simulink library "miniview_lib"  (Simulink 5.1)
undefined symbols (not defined in the file or in its folder): DN, miniview_string_xfer_page0, miniview_string_xfer_page1, miniview_string_xfer_page2, ptr, UP
libraries: simulink x33, MotoHawk_lib x17, miniview_lib x8
settings Model: LastModifiedBy=Chris_Doyle  ProdHWDeviceType=Microprocessor

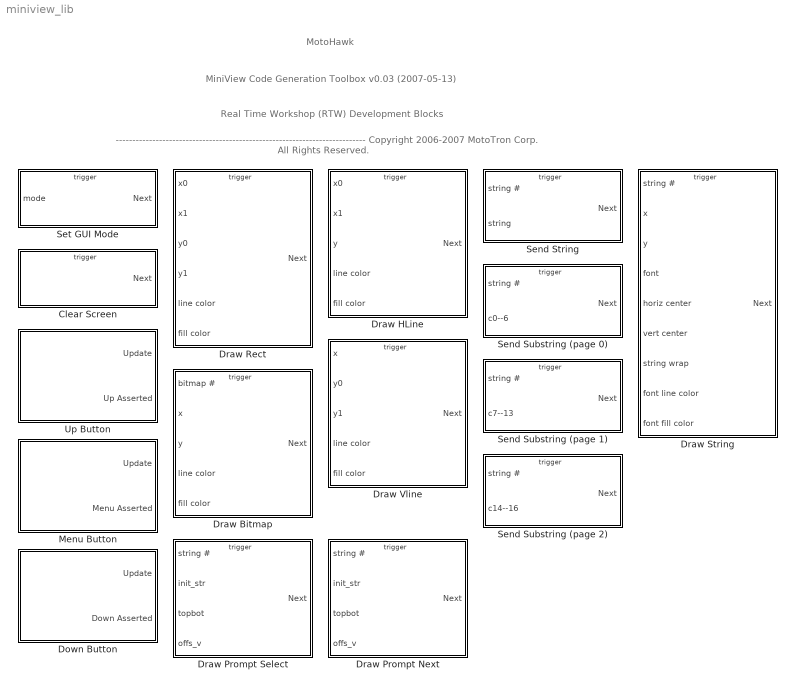
== system miniview_lib ==
  note: MotoHawk
  note: ---------------------------------------------------------------------------
      | Copyright 2006-2007 MotoTron Corp.  All Rights Reserved.
  note: Real Time Workshop (RTW)
      | Development Blocks
  note: MiniView Code Generation Toolbox v0.03 (2007-05-13)
  Clear Screen : Subsystem  mask(MotoHawk MiniView Clear Screen){miniview_CAN_channel=2}
      mask prompts: miniview_CAN_channel "Physical CAN Channel"
      mask help: MotoHawk MiniView Clear Screen
      mask Display: disp(['\nMiniView\nClear Screen\nChannel:  CAN_' num2str(miniview_CAN_channel)])
  Down Button : Subsystem  mask(MotoHawk MiniView Down Button){miniview_CAN_channel=2}
      mask prompts: miniview_CAN_channel "Physical CAN Channel"
      mask help: MotoHawk MiniView Down Button
      mask Display: disp(['MiniView "Down" Button\nChannel:  CAN_' num2str(miniview_CAN_channel)])
  Draw Bitmap : Subsystem  mask(MotoHawk MiniView Draw Bitmap){miniview_CAN_channel=2}
      mask prompts: miniview_CAN_channel "Physical CAN Channel"
      mask help:
      | MotoHawk MiniView Draw Bitmap
      | 0:  "Dialog"
      | 1:  small down-arrow
      | 2:  large down-arrow
      | 3:  selector down-arrow
      | 4:  selector up-arrow
      mask Display: disp(['MiniView\nDraw Bitmap\nChannel:  CAN_' num2str(miniview_CAN_channel) '\n\n\n\n'])
  Draw HLine : Subsystem  mask(MotoHawk MiniView Draw Horizontal Line){miniview_CAN_channel=2}
      mask prompts: miniview_CAN_channel "Physical CAN Channel"
      mask help: MotoHawk MiniView Draw Horizontal Line
      mask Display: disp(['MiniView\nDraw Horiz Line\nChannel:  CAN_' num2str(miniview_CAN_channel) '\n\n\n\n'])
  Draw Prompt Next : Subsystem  mask(MotoHawk MiniView Draw Prompt Next){miniview_CAN_channel=2}
      mask prompts: miniview_CAN_channel "Physical CAN Channel"
      mask help:
      | MotoHawk MiniView Draw Prompt Next
      |
      | string # (0 to 15):  which string buffer to use.
      |
      | init_str (F,T):  when TRUE, initialize string buffer in gauge (by sending CAN message).  must be done first time prompt is drawn, and whenever buffer has been changed.
      |
      | topbot (F,T):  when FALSE, prompt at "top" position; when TRUE, prompt at "bottom" position.
      |
      | offs_v (0 to 55 when topbot is FALSE, otherwise 0):  vertical offset (downwards) for prompt from "top" position.
      mask Display: disp(['\nDraw\nPrompt\n[up]NEXT[dn]\nChannel:  CAN_' num2str(miniview_CAN_channel)])
  Draw Prompt Select : Subsystem  mask(MotoHawk MiniView Draw Prompt Select){miniview_CAN_channel=2}
      mask prompts: miniview_CAN_channel "Physical CAN Channel"
      mask help:
      | MotoHawk MiniView Draw Prompt Select
      |
      | string # (0 to 15):  which string buffer to use.
      |
      | init_str (F,T):  when TRUE, initialize string buffer in gauge (by sending CAN message).  must be done first time prompt is drawn, and whenever buffer has been changed.
      |
      | topbot (F,T):  when FALSE, prompt at "top" position; when TRUE, prompt at "bottom" position.
      |
      | offs_v (0 to 55 when topbot is FALSE, otherwise 0):  vertical offset (downwards) for prompt from "top" position.
      mask Display: disp(['\nDraw\nPrompt\n[up]SEL[dn]\nChannel:  CAN_' num2str(miniview_CAN_channel)])
  Draw Rect : Subsystem  mask(MotoHawk MiniView Draw Rectangle){miniview_CAN_channel=2}
      mask prompts: miniview_CAN_channel "Physical CAN Channel"
      mask help: MotoHawk MiniView Draw Rectangle
      mask Display: disp(['MiniView\nDraw Rectangle\nChannel:  CAN_' num2str(miniview_CAN_channel) '\n\n\n\n'])
  Draw String : Subsystem  mask(MotoHawk MiniView Draw String){miniview_CAN_channel=2}
      mask prompts: miniview_CAN_channel "Physical CAN Channel"
      mask help:
      | MotoHawk MiniView Draw String
      |
      | Draw string (#0 to #15) previously sent to gauge using "Send String"
      | or "Send Substring (Page 0/1/2)" blocks.
      |
      | Comment:  "Font Fill Color" input is ignored.
      mask Display: disp(['MiniView\nDraw String\nChannel:  CAN_' num2str(miniview_CAN_channel) '\n\n\n\n'])
  Draw Vline : Subsystem  mask(MotoHawk MiniView Draw Vertical Line){miniview_CAN_channel=2}
      mask prompts: miniview_CAN_channel "Physical CAN Channel"
      mask help: MotoHawk MiniView Draw Vertical Line
      mask Display: disp(['MiniView\nDraw Vert Line\nChannel:  CAN_' num2str(miniview_CAN_channel) '\n\n\n\n'])
  Menu Button : Subsystem  mask(MotoHawk MiniView Menu Button){miniview_CAN_channel=2}
      mask prompts: miniview_CAN_channel "Physical CAN Channel"
      mask help: MotoHawk MiniView Menu Button
      mask Display: disp(['MiniView "Menu" Button\nChannel:  CAN_' num2str(miniview_CAN_channel)])
  Send String : Subsystem  mask(MotoHawk MiniView Send String){miniview_CAN_channel=2}
      mask prompts: miniview_CAN_channel "Physical CAN Channel"
      mask help:
      | MotoHawk MiniView Send String
      |
      | Send string (#0 to #15) to gauge.
      mask Display: disp(['MiniView\nSend String\nChannel:  CAN_' num2str(miniview_CAN_channel)])
  Send Substring (page 0) : Subsystem  mask(MotoHawk MiniView Send String (Page 0)){miniview_CAN_channel=2}
      mask prompts: miniview_CAN_channel "Physical CAN Channel"
      mask help:
      | MotoHawk MiniView Send String (Page 0)
      |
      | Send first seven characters (0 to 6) of string (#0 to #15) to gauge.
      |
      | Before using a string, all three pages (0/1/2) must be sent using either "Send String" block to send the entire string at once, or by sending each page using "Send Substring (Page 0/1/2)" blocks.
      |
      | The "Send Substring (Page 0/1/2)" blocks may also be used to modify a previously-sent string.
      mask Display: disp(['MiniView\nSend Substr Pg 0\nChannel:  CAN_' num2str(miniview_CAN_channel)])
  Send Substring (page 1) : Subsystem  mask(MotoHawk MiniView Send String (Page 1)){miniview_CAN_channel=2}
      mask prompts: miniview_CAN_channel "Physical CAN Channel"
      mask help:
      | MotoHawk MiniView Send String (Page 1)
      |
      | Send middle seven characters (7 to 13) of string (#0 to #15) to gauge.
      |
      | Before using a string, all three pages (0/1/2) must be sent using either "Send String" block to send the entire string at once, or by sending each page using "Send Substring (Page 0/1/2)" blocks.
      |
      | The "Send Substring (Page 0/1/2)" blocks may also be used to modify a previously-sent string.
      mask Display: disp(['MiniView\nSend Substr Pg 1\nChannel:  CAN_' num2str(miniview_CAN_channel)])
  Send Substring (page 2) : Subsystem  mask(MotoHawk MiniView Send String (Page 2)){miniview_CAN_channel=2}
      mask prompts: miniview_CAN_channel "Physical CAN Channel"
      mask help:
      | MotoHawk MiniView Send String (Page 2)
      |
      | Send last three characters (14 to 16) of string (#0 to #15) to gauge.
      |
      | Before using a string, all three pages (0/1/2) must be sent using either "Send String" block to send the entire string at once, or by sending each page using "Send Substring (Page 0/1/2)" blocks.
      |
      | The "Send Substring (Page 0/1/2)" blocks may also be used to modify a previously-sent string.
      mask Display: disp(['MiniView\nSend Substr Pg 2\nChannel:  CAN_' num2str(miniview_CAN_channel)])
  Set GUI Mode : Subsystem  mask(MotoHawk MiniView Set GUI Mode){miniview_CAN_channel=2}
      mask prompts: miniview_CAN_channel "Physical CAN Channel"
      mask help: MotoHawk MiniView Set GUI Mode
      mask Display: disp(['\nMiniView\nSet GUI Mode\nChannel:  CAN_' num2str(miniview_CAN_channel)])
  Up Button : Subsystem  mask(MotoHawk MiniView Up Button){miniview_CAN_channel=2}
      mask prompts: miniview_CAN_channel "Physical CAN Channel"
      mask help: MotoHawk MiniView Up Button
      mask Display: disp(['MiniView "Up" Button\nChannel:  CAN_' num2str(miniview_CAN_channel)])

== system miniview_lib/Clear Screen ==
  Trigger : TriggerPort  TriggerType=function-call
  Clear Screen : Subsystem
  Demux : Demux  Orientation=down  Outputs=2
  Function-Call Generator : simulink/Ports & Subsystems/Function-Call Generator  sample_time=-1  numberOfIterations=1
  Next : Outport
  wires:
  Demux/2 -> Next/1
  Function-Call Generator/1 -> Demux/1
  Demux/1 -> Clear Screen/Trigger

== system miniview_lib/Down Button ==
  CAN Receive Slot Trigger : MotoHawk_lib/CAN Blocks/CAN Receive Slot Trigger  Tag=Trigger  Orientation=down  slot='miniview_button_down'  inherited=on  function_name=Trigger_CAN_Slot_miniview_button_down_669p0004
  Demux : Demux  Orientation=down  Outputs=2
  Subsystem : Subsystem
  Terminator : Terminator
  Update : Outport
  Down Asserted : Outport  Port=2
  wires:
  Subsystem/1(Out1) -> Down Asserted/1
  Demux/1 -> Subsystem/Trigger
  CAN Receive Slot Trigger/1 -> Demux/1
  Demux/2 -> Update/1
  Subsystem/2(Out2) -> Terminator/1

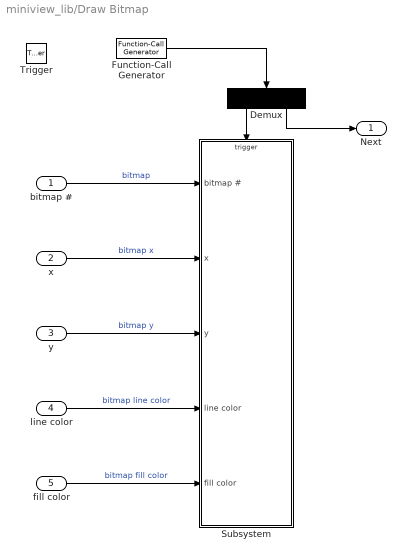
== system miniview_lib/Draw Bitmap ==
  bitmap # : Inport
  x : Inport  Port=2
  y : Inport  Port=3
  line color : Inport  Port=4
  fill color : Inport  Port=5
  Trigger : TriggerPort  TriggerType=function-call
  Demux : Demux  Orientation=down  Outputs=2
  Function-Call Generator : simulink/Ports & Subsystems/Function-Call Generator  sample_time=-1  numberOfIterations=1
  Subsystem : Subsystem
  Next : Outport
  wires:
  bitmap #/1 -> Subsystem/1(bitmap #)  "bitmap"
  x/1 -> Subsystem/2(x)  "bitmap x"
  y/1 -> Subsystem/3(y)  "bitmap y"
  line color/1 -> Subsystem/4(line color)  "bitmap line color"
  fill color/1 -> Subsystem/5(fill color)  "bitmap fill color"
  Demux/1 -> Subsystem/Trigger
  Function-Call Generator/1 -> Demux/1
  Demux/2 -> Next/1

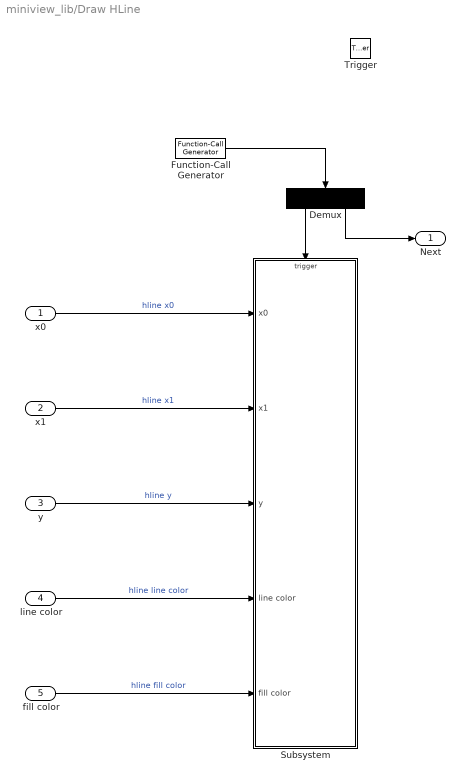
== system miniview_lib/Draw HLine ==
  x0 : Inport
  x1 : Inport  Port=2
  y : Inport  Port=3
  line color : Inport  Port=4
  fill color : Inport  Port=5
  Trigger : TriggerPort  TriggerType=function-call
  Demux : Demux  Orientation=down  Outputs=2
  Function-Call Generator : simulink/Ports & Subsystems/Function-Call Generator  sample_time=-1  numberOfIterations=1
  Subsystem : Subsystem
  Next : Outport
  wires:
  x0/1 -> Subsystem/1(x0)  "hline x0"
  x1/1 -> Subsystem/2(x1)  "hline x1"
  y/1 -> Subsystem/3(y)  "hline y"
  line color/1 -> Subsystem/4(line color)  "hline line color"
  fill color/1 -> Subsystem/5(fill color)  "hline fill color"
  Demux/1 -> Subsystem/Trigger
  Function-Call Generator/1 -> Demux/1
  Demux/2 -> Next/1

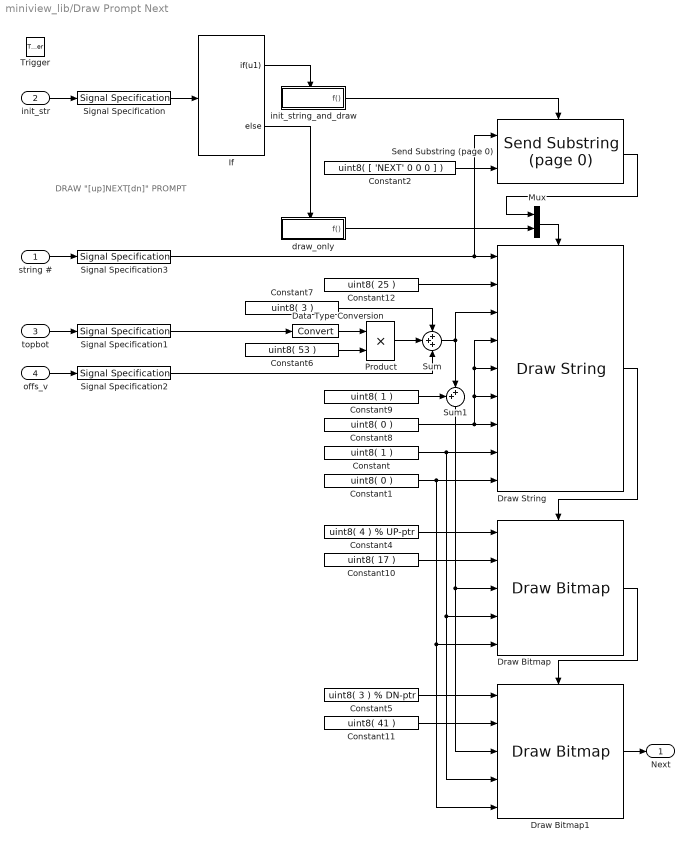
== system miniview_lib/Draw Prompt Next ==
  note: DRAW
      | "[up]NEXT[dn]"
      | PROMPT
  string # : Inport
  init_str : Inport  Port=2
  topbot : Inport  Port=3
  offs_v : Inport  Port=4
  Trigger : TriggerPort  TriggerType=function-call
  Constant : Constant  Value=uint8( 1 )
  Constant1 : Constant  Value=uint8( 0 )
  Constant10 : Constant  Value=uint8( 17 )
  Constant11 : Constant  Value=uint8( 41 )
  Constant12 : Constant  Value=uint8( 25 )
  Constant2 : Constant  Value=uint8( [ 'NEXT' 0 0 0 ] )
  Constant4 : Constant  Value=uint8( 4 ) % UP-ptr
  Constant5 : Constant  Value=uint8( 3 ) % DN-ptr
  Constant6 : Constant  Value=uint8( 53 )
  Constant7 : Constant  Value=uint8( 3 )
  Constant8 : Constant  Value=uint8( 0 )
  Constant9 : Constant  Value=uint8( 1 )
  Data Type Conversion : DataTypeConversion
  Draw Bitmap : miniview_lib/Draw Bitmap  miniview_CAN_channel=miniview_CAN_channel
  Draw Bitmap1 : miniview_lib/Draw Bitmap  miniview_CAN_channel=miniview_CAN_channel
  Draw String : miniview_lib/Draw String  miniview_CAN_channel=miniview_CAN_channel
  If : If  IfExpression=u1
  Mux : Mux  Inputs=2
  Product : Product  OutDataTypeMode=uint8  RndMeth=Zero  InputSameDT=on
  Send Substring (page 0) : miniview_lib/Send Substring (page 0)  miniview_CAN_channel=miniview_CAN_channel
  Signal Specification : simulink/Signal Attributes/Signal Specification  D=1  Ts=-1  DataType=boolean  OutDataType=sfix(16)  OutScaling=2^0
      settings: SignalType=auto  SamplingMode=auto
  Signal Specification1 : simulink/Signal Attributes/Signal Specification  D=1  Ts=-1  DataType=boolean  OutDataType=sfix(16)  OutScaling=2^0
      settings: SignalType=auto  SamplingMode=auto
  Signal Specification2 : simulink/Signal Attributes/Signal Specification  D=1  Ts=-1  DataType=uint8  OutDataType=sfix(16)  OutScaling=2^0
      settings: SignalType=auto  SamplingMode=auto
  Signal Specification3 : simulink/Signal Attributes/Signal Specification  D=1  Ts=-1  DataType=uint8  OutDataType=sfix(16)  OutScaling=2^0
      settings: SignalType=auto  SamplingMode=auto
  Sum : Sum  Inputs=+++  RndMeth=Zero  InputSameDT=on
  Sum1 : Sum  Orientation=down  Inputs=++|  RndMeth=Zero  InputSameDT=on
  draw_only : Subsystem
  init_string_and_draw : Subsystem
  Next : Outport
  wires:
  Signal Specification3/1 -> Draw String/1, Send Substring (page 0)/1
  string #/1 -> Signal Specification3/1
  Signal Specification/1 -> If/1
  draw_only/1(f()) -> Mux/2
  init_string_and_draw/1(f()) -> Send Substring (page 0)/Trigger
  If/2 -> draw_only/Action
  If/1 -> init_string_and_draw/Action
  Mux/1 -> Draw String/Trigger
  Sum/1 -> Sum1/2, Draw String/3
  Constant6/1 -> Product/2
  Constant10/1 -> Draw Bitmap/2
  Constant11/1 -> Draw Bitmap1/2
  Constant12/1 -> Draw String/2
  Constant9/1 -> Sum1/1
  Sum1/1 -> Draw Bitmap/3, Draw Bitmap1/3
  Constant8/1 -> Draw String/4, Draw String/5, Draw String/6, Draw String/7
  Signal Specification2/1 -> Sum/3
  Product/1 -> Sum/2
  Constant7/1 -> Sum/1
  Data Type Conversion/1 -> Product/1
  Signal Specification1/1 -> Data Type Conversion/1
  offs_v/1 -> Signal Specification2/1
  topbot/1 -> Signal Specification1/1
  init_str/1 -> Signal Specification/1
  Draw Bitmap/1 -> Draw Bitmap1/Trigger
  Send Substring (page 0)/1 -> Mux/1
  Draw String/1 -> Draw Bitmap/Trigger
  Draw Bitmap1/1 -> Next/1
  Constant4/1 -> Draw Bitmap/1
  Constant5/1 -> Draw Bitmap1/1
  Constant2/1 -> Send Substring (page 0)/2
  Constant1/1 -> Draw String/9, Draw Bitmap1/5, Draw Bitmap/5
  Constant/1 -> Draw String/8, Draw Bitmap1/4, Draw Bitmap/4

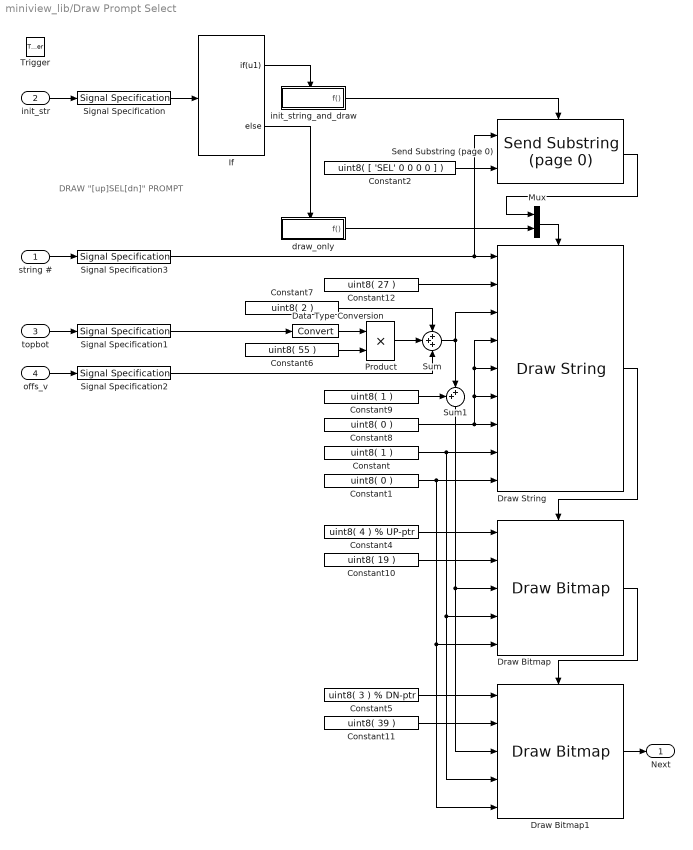
== system miniview_lib/Draw Prompt Select ==
  note: DRAW
      | "[up]SEL[dn]"
      | PROMPT
  string # : Inport
  init_str : Inport  Port=2
  topbot : Inport  Port=3
  offs_v : Inport  Port=4
  Trigger : TriggerPort  TriggerType=function-call
  Constant : Constant  Value=uint8( 1 )
  Constant1 : Constant  Value=uint8( 0 )
  Constant10 : Constant  Value=uint8( 19 )
  Constant11 : Constant  Value=uint8( 39 )
  Constant12 : Constant  Value=uint8( 27 )
  Constant2 : Constant  Value=uint8( [ 'SEL' 0 0 0 0 ] )
  Constant4 : Constant  Value=uint8( 4 ) % UP-ptr
  Constant5 : Constant  Value=uint8( 3 ) % DN-ptr
  Constant6 : Constant  Value=uint8( 55 )
  Constant7 : Constant  Value=uint8( 2 )
  Constant8 : Constant  Value=uint8( 0 )
  Constant9 : Constant  Value=uint8( 1 )
  Data Type Conversion : DataTypeConversion
  Draw Bitmap : miniview_lib/Draw Bitmap  miniview_CAN_channel=miniview_CAN_channel
  Draw Bitmap1 : miniview_lib/Draw Bitmap  miniview_CAN_channel=miniview_CAN_channel
  Draw String : miniview_lib/Draw String  miniview_CAN_channel=miniview_CAN_channel
  If : If  IfExpression=u1
  Mux : Mux  Inputs=2
  Product : Product  OutDataTypeMode=uint8  RndMeth=Zero  InputSameDT=on
  Send Substring (page 0) : miniview_lib/Send Substring (page 0)  miniview_CAN_channel=miniview_CAN_channel
  Signal Specification : simulink/Signal Attributes/Signal Specification  D=1  Ts=-1  DataType=boolean  OutDataType=sfix(16)  OutScaling=2^0
      settings: SignalType=auto  SamplingMode=auto
  Signal Specification1 : simulink/Signal Attributes/Signal Specification  D=1  Ts=-1  DataType=boolean  OutDataType=sfix(16)  OutScaling=2^0
      settings: SignalType=auto  SamplingMode=auto
  Signal Specification2 : simulink/Signal Attributes/Signal Specification  D=1  Ts=-1  DataType=uint8  OutDataType=sfix(16)  OutScaling=2^0
      settings: SignalType=auto  SamplingMode=auto
  Signal Specification3 : simulink/Signal Attributes/Signal Specification  D=1  Ts=-1  DataType=uint8  OutDataType=sfix(16)  OutScaling=2^0
      settings: SignalType=auto  SamplingMode=auto
  Sum : Sum  Inputs=+++  RndMeth=Zero  InputSameDT=on
  Sum1 : Sum  Orientation=down  Inputs=++|  RndMeth=Zero  InputSameDT=on
  draw_only : Subsystem
  init_string_and_draw : Subsystem
  Next : Outport
  wires:
  Constant/1 -> Draw Bitmap/4, Draw Bitmap1/4, Draw String/8
  Constant1/1 -> Draw Bitmap/5, Draw Bitmap1/5, Draw String/9
  Constant2/1 -> Send Substring (page 0)/2
  Constant5/1 -> Draw Bitmap1/1
  Constant4/1 -> Draw Bitmap/1
  Draw Bitmap1/1 -> Next/1
  Draw String/1 -> Draw Bitmap/Trigger
  Send Substring (page 0)/1 -> Mux/1
  Draw Bitmap/1 -> Draw Bitmap1/Trigger
  init_str/1 -> Signal Specification/1
  topbot/1 -> Signal Specification1/1
  offs_v/1 -> Signal Specification2/1
  Signal Specification1/1 -> Data Type Conversion/1
  Data Type Conversion/1 -> Product/1
  Constant7/1 -> Sum/1
  Product/1 -> Sum/2
  Signal Specification2/1 -> Sum/3
  Constant8/1 -> Draw String/7, Draw String/6, Draw String/5, Draw String/4
  Sum1/1 -> Draw Bitmap1/3, Draw Bitmap/3
  Constant9/1 -> Sum1/1
  Constant12/1 -> Draw String/2
  Constant11/1 -> Draw Bitmap1/2
  Constant10/1 -> Draw Bitmap/2
  Constant6/1 -> Product/2
  Sum/1 -> Draw String/3, Sum1/2
  Mux/1 -> Draw String/Trigger
  If/1 -> init_string_and_draw/Action
  If/2 -> draw_only/Action
  init_string_and_draw/1(f()) -> Send Substring (page 0)/Trigger
  draw_only/1(f()) -> Mux/2
  Signal Specification/1 -> If/1
  string #/1 -> Signal Specification3/1
  Signal Specification3/1 -> Send Substring (page 0)/1, Draw String/1

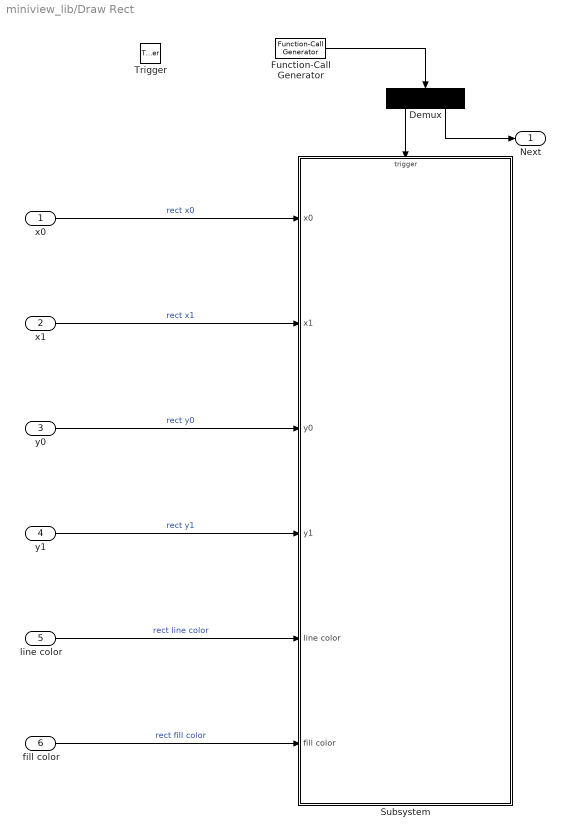
== system miniview_lib/Draw Rect ==
  x0 : Inport
  x1 : Inport  Port=2
  y0 : Inport  Port=3
  y1 : Inport  Port=4
  line color : Inport  Port=5
  fill color : Inport  Port=6
  Trigger : TriggerPort  TriggerType=function-call
  Demux : Demux  Orientation=down  Outputs=2
  Function-Call Generator : simulink/Ports & Subsystems/Function-Call Generator  sample_time=-1  numberOfIterations=1
  Subsystem : Subsystem
  Next : Outport
  wires:
  x0/1 -> Subsystem/1(x0)  "rect x0"
  x1/1 -> Subsystem/2(x1)  "rect x1"
  y0/1 -> Subsystem/3(y0)  "rect y0"
  y1/1 -> Subsystem/4(y1)  "rect y1"
  line color/1 -> Subsystem/5(line color)  "rect line color"
  fill color/1 -> Subsystem/6(fill color)  "rect fill color"
  Demux/1 -> Subsystem/Trigger
  Function-Call Generator/1 -> Demux/1
  Demux/2 -> Next/1

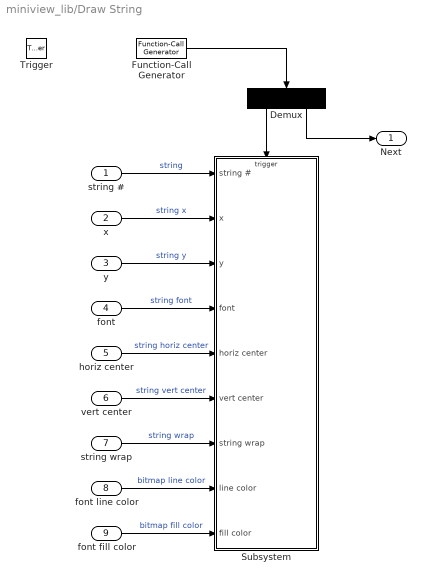
== system miniview_lib/Draw String ==
  string # : Inport
  x : Inport  Port=2
  y : Inport  Port=3
  font : Inport  Port=4
  horiz center : Inport  Port=5
  vert center : Inport  Port=6
  string wrap : Inport  Port=7
  font line color : Inport  Port=8
  font fill color : Inport  Port=9
  Trigger : TriggerPort  TriggerType=function-call
  Demux : Demux  Orientation=down  Outputs=2
  Function-Call Generator : simulink/Ports & Subsystems/Function-Call Generator  sample_time=-1  numberOfIterations=1
  Subsystem : Subsystem
  Next : Outport
  wires:
  string #/1 -> Subsystem/1(string #)  "string"
  x/1 -> Subsystem/2(x)  "string x"
  y/1 -> Subsystem/3(y)  "string y"
  font/1 -> Subsystem/4(font)  "string font"
  horiz center/1 -> Subsystem/5(horiz center)  "string horiz center"
  vert center/1 -> Subsystem/6(vert center)  "string vert center"
  string wrap/1 -> Subsystem/7(string wrap)  "string wrap"
  font line color/1 -> Subsystem/8(line color)  "bitmap line color"
  font fill color/1 -> Subsystem/9(fill color)  "bitmap fill color"
  Demux/1 -> Subsystem/Trigger
  Function-Call Generator/1 -> Demux/1
  Demux/2 -> Next/1

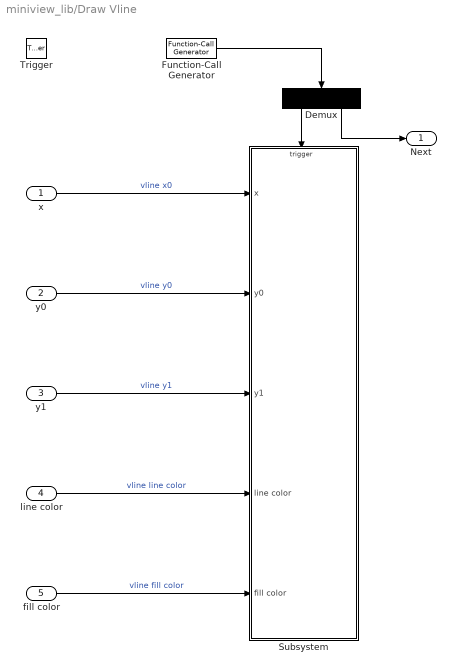
== system miniview_lib/Draw Vline ==
  x : Inport
  y0 : Inport  Port=2
  y1 : Inport  Port=3
  line color : Inport  Port=4
  fill color : Inport  Port=5
  Trigger : TriggerPort  TriggerType=function-call
  Demux : Demux  Orientation=down  Outputs=2
  Function-Call Generator : simulink/Ports & Subsystems/Function-Call Generator  sample_time=-1  numberOfIterations=1
  Subsystem : Subsystem
  Next : Outport
  wires:
  x/1 -> Subsystem/1(x)  "vline x0"
  y0/1 -> Subsystem/2(y0)  "vline y0"
  y1/1 -> Subsystem/3(y1)  "vline y1"
  line color/1 -> Subsystem/4(line color)  "vline line color"
  fill color/1 -> Subsystem/5(fill color)  "vline fill color"
  Demux/1 -> Subsystem/Trigger
  Function-Call Generator/1 -> Demux/1
  Demux/2 -> Next/1

== system miniview_lib/Menu Button ==
  CAN Receive Slot Trigger : MotoHawk_lib/CAN Blocks/CAN Receive Slot Trigger  Tag=Trigger  Orientation=down  slot='miniview_button_menu'  inherited=on  function_name=Trigger_CAN_Slot_miniview_button_menu_667p0002
  Demux : Demux  Orientation=down  Outputs=2
  Subsystem : Subsystem
  Terminator : Terminator
  Update : Outport
  Menu Asserted : Outport  Port=2
  wires:
  Subsystem/2(Out2) -> Terminator/1
  Demux/2 -> Update/1
  CAN Receive Slot Trigger/1 -> Demux/1
  Demux/1 -> Subsystem/Trigger
  Subsystem/1(Out1) -> Menu Asserted/1

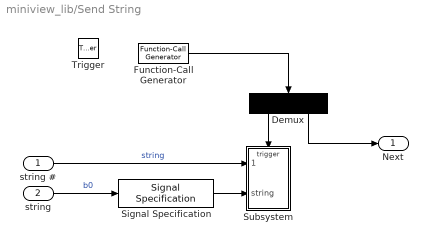
== system miniview_lib/Send String ==
  string # : Inport
  string : Inport  Port=2
  Trigger : TriggerPort  TriggerType=function-call
  Demux : Demux  Orientation=down  Outputs=2
  Function-Call Generator : simulink/Ports & Subsystems/Function-Call Generator  sample_time=-1  numberOfIterations=1
  Signal Specification : simulink/Signal Attributes/Signal Specification  D=18  Ts=-1  DataType=uint8  OutDataType=sfix(16)  OutScaling=2^0
      settings: SignalType=auto  SamplingMode=auto
  Subsystem : Subsystem
  Next : Outport
  wires:
  string #/1 -> Subsystem/1(string #)  "string"
  string/1 -> Signal Specification/1  "b0"
  Demux/1 -> Subsystem/Trigger
  Function-Call Generator/1 -> Demux/1
  Demux/2 -> Next/1
  Signal Specification/1 -> Subsystem/2(string)

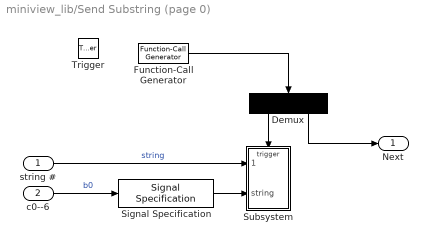
== system miniview_lib/Send Substring (page 0) ==
  string # : Inport
  c0--6 : Inport  Port=2
  Trigger : TriggerPort  TriggerType=function-call
  Demux : Demux  Orientation=down  Outputs=2
  Function-Call Generator : simulink/Ports & Subsystems/Function-Call Generator  sample_time=-1  numberOfIterations=1
  Signal Specification : simulink/Signal Attributes/Signal Specification  D=7  Ts=-1  DataType=uint8  OutDataType=sfix(16)  OutScaling=2^0
      settings: SignalType=auto  SamplingMode=auto
  Subsystem : Subsystem
  Next : Outport
  wires:
  Signal Specification/1 -> Subsystem/2(string)
  Demux/2 -> Next/1
  Function-Call Generator/1 -> Demux/1
  Demux/1 -> Subsystem/Trigger
  c0--6/1 -> Signal Specification/1  "b0"
  string #/1 -> Subsystem/1(string #)  "string"

== system miniview_lib/Send Substring (page 1) ==
  string # : Inport
  c7--13 : Inport  Port=2
  Trigger : TriggerPort  TriggerType=function-call
  Demux : Demux  Orientation=down  Outputs=2
  Function-Call Generator : simulink/Ports & Subsystems/Function-Call Generator  sample_time=-1  numberOfIterations=1
  Signal Specification : simulink/Signal Attributes/Signal Specification  D=7  Ts=-1  DataType=uint8  OutDataType=sfix(16)  OutScaling=2^0
      settings: SignalType=auto  SamplingMode=auto
  Subsystem : Subsystem
  Next : Outport
  wires:
  string #/1 -> Subsystem/1(string #)  "string"
  c7--13/1 -> Signal Specification/1  "b0"
  Demux/1 -> Subsystem/Trigger
  Function-Call Generator/1 -> Demux/1
  Demux/2 -> Next/1
  Signal Specification/1 -> Subsystem/2(string)

== system miniview_lib/Send Substring (page 2) ==
  string # : Inport
  c14--16 : Inport  Port=2
  Trigger : TriggerPort  TriggerType=function-call
  Demux : Demux  Orientation=down  Outputs=2
  Function-Call Generator : simulink/Ports & Subsystems/Function-Call Generator  sample_time=-1  numberOfIterations=1
  Signal Specification : simulink/Signal Attributes/Signal Specification  D=3  Ts=-1  DataType=uint8  OutDataType=sfix(16)  OutScaling=2^0
      settings: SignalType=auto  SamplingMode=auto
  Subsystem : Subsystem
  Next : Outport
  wires:
  string #/1 -> Subsystem/1(string #)  "string"
  c14--16/1 -> Signal Specification/1  "b0"
  Demux/1 -> Subsystem/Trigger
  Function-Call Generator/1 -> Demux/1
  Demux/2 -> Next/1
  Signal Specification/1 -> Subsystem/2(string)

== system miniview_lib/Set GUI Mode ==
  mode : Inport
  Trigger : TriggerPort  TriggerType=function-call
  Demux : Demux  Orientation=down  Outputs=2
  Function-Call Generator : simulink/Ports & Subsystems/Function-Call Generator  sample_time=-1  numberOfIterations=1
  Subsystem : Subsystem
  Next : Outport
  wires:
  mode/1 -> Subsystem/1(mode)  "mode"
  Demux/1 -> Subsystem/Trigger
  Function-Call Generator/1 -> Demux/1
  Demux/2 -> Next/1

== system miniview_lib/Up Button ==
  CAN Receive Slot Trigger : MotoHawk_lib/CAN Blocks/CAN Receive Slot Trigger  Tag=Trigger  Orientation=down  slot='miniview_button_up'  inherited=on  function_name=Trigger_CAN_Slot_miniview_button_up_644p0001
  Demux : Demux  Orientation=down  Outputs=2
  Subsystem : Subsystem
  Terminator : Terminator
  Update : Outport
  Up Asserted : Outport  Port=2
  wires:
  Subsystem/1(Out1) -> Up Asserted/1
  Demux/1 -> Subsystem/Trigger
  CAN Receive Slot Trigger/1 -> Demux/1
  Demux/2 -> Update/1
  Subsystem/2(Out2) -> Terminator/1

== system miniview_lib/Clear Screen/Clear Screen ==
  Trigger : TriggerPort  TriggerType=function-call
  Send CAN Messages : MotoHawk_lib/CAN Blocks/Send CAN Messages  bus=miniview_CAN_channel  msgl=miniview_clear_screen  pace=-1  labelwires=off

== system miniview_lib/Down Button/Subsystem ==
  Trigger : TriggerPort  TriggerType=function-call
  Read CAN Message : MotoHawk_lib/CAN Blocks/Read CAN Message  bus=miniview_CAN_channel  msg=miniview_button_down  queue=1  slot='miniview_button_down'  valid=off  stale=off  labelwires=on
  Signal Specification : simulink/Signal Attributes/Signal Specification  D=-1  Ts=-1  DataType=boolean  OutDataType=sfix(16)  OutScaling=2^0
      settings: SignalType=auto  SamplingMode=auto
  Signal Specification1 : simulink/Signal Attributes/Signal Specification  D=-1  Ts=-1  DataType=uint8  OutDataType=sfix(16)  OutScaling=2^0
      settings: SignalType=auto  SamplingMode=auto
  Out1 : Outport
  Out2 : Outport  Port=2
  wires:
  Read CAN Message/1 -> Signal Specification/1  "down asserted"
  Read CAN Message/2 -> Signal Specification1/1  "down count"
  Signal Specification/1 -> Out1/1  "down asserted"
  Signal Specification1/1 -> Out2/1  "down count"

== system miniview_lib/Draw Bitmap/Subsystem ==
  bitmap # : Inport
  x : Inport  Port=2
  y : Inport  Port=3
  line color : Inport  Port=4
  fill color : Inport  Port=5
  Trigger : TriggerPort  TriggerType=function-call
  Send CAN Messages : MotoHawk_lib/CAN Blocks/Send CAN Messages  bus=miniview_CAN_channel  msgl=miniview_draw_bitmap  pace=-1  labelwires=on
  wires:
  fill color/1 -> Send CAN Messages/5  "fill color"
  line color/1 -> Send CAN Messages/4  "line color"
  bitmap #/1 -> Send CAN Messages/1  "bitmap #"
  x/1 -> Send CAN Messages/2  "bitmap x"
  y/1 -> Send CAN Messages/3  "bitmap y"

== system miniview_lib/Draw HLine/Subsystem ==
  x0 : Inport
  x1 : Inport  Port=2
  y : Inport  Port=3
  line color : Inport  Port=4
  fill color : Inport  Port=5
  Trigger : TriggerPort  TriggerType=function-call
  Send CAN Messages : MotoHawk_lib/CAN Blocks/Send CAN Messages  bus=miniview_CAN_channel  msgl=miniview_draw_hline  pace=-1  labelwires=on
  wires:
  y/1 -> Send CAN Messages/3  "hline y"
  x1/1 -> Send CAN Messages/2  "hline x1"
  x0/1 -> Send CAN Messages/1  "hline x0"
  line color/1 -> Send CAN Messages/4  "line color"
  fill color/1 -> Send CAN Messages/5  "fill color"

== system miniview_lib/Draw Prompt Next/draw_only ==
  Action Port : ActionPort
  Function-Call Generator : simulink/Ports & Subsystems/Function-Call Generator  sample_time=-1  numberOfIterations=1
  f() : Outport
  wires:
  Function-Call Generator/1 -> f()/1

== system miniview_lib/Draw Prompt Next/init_string_and_draw ==
  Action Port : ActionPort
  Function-Call Generator : simulink/Ports & Subsystems/Function-Call Generator  sample_time=-1  numberOfIterations=1
  f() : Outport
  wires:
  Function-Call Generator/1 -> f()/1

== system miniview_lib/Draw Prompt Select/draw_only ==
  Action Port : ActionPort
  Function-Call Generator : simulink/Ports & Subsystems/Function-Call Generator  sample_time=-1  numberOfIterations=1
  f() : Outport
  wires:
  Function-Call Generator/1 -> f()/1

== system miniview_lib/Draw Prompt Select/init_string_and_draw ==
  Action Port : ActionPort
  Function-Call Generator : simulink/Ports & Subsystems/Function-Call Generator  sample_time=-1  numberOfIterations=1
  f() : Outport
  wires:
  Function-Call Generator/1 -> f()/1

== system miniview_lib/Draw Rect/Subsystem ==
  x0 : Inport
  x1 : Inport  Port=2
  y0 : Inport  Port=3
  y1 : Inport  Port=4
  line color : Inport  Port=5
  fill color : Inport  Port=6
  Trigger : TriggerPort  TriggerType=function-call
  Send CAN Messages : MotoHawk_lib/CAN Blocks/Send CAN Messages  bus=miniview_CAN_channel  msgl=miniview_draw_rectangle  pace=-1  labelwires=on
  wires:
  x0/1 -> Send CAN Messages/1  "rect x0"
  x1/1 -> Send CAN Messages/2  "rect x1"
  y0/1 -> Send CAN Messages/3  "rect y0"
  y1/1 -> Send CAN Messages/4  "rect y1"
  line color/1 -> Send CAN Messages/5  "line color"
  fill color/1 -> Send CAN Messages/6  "fill color"

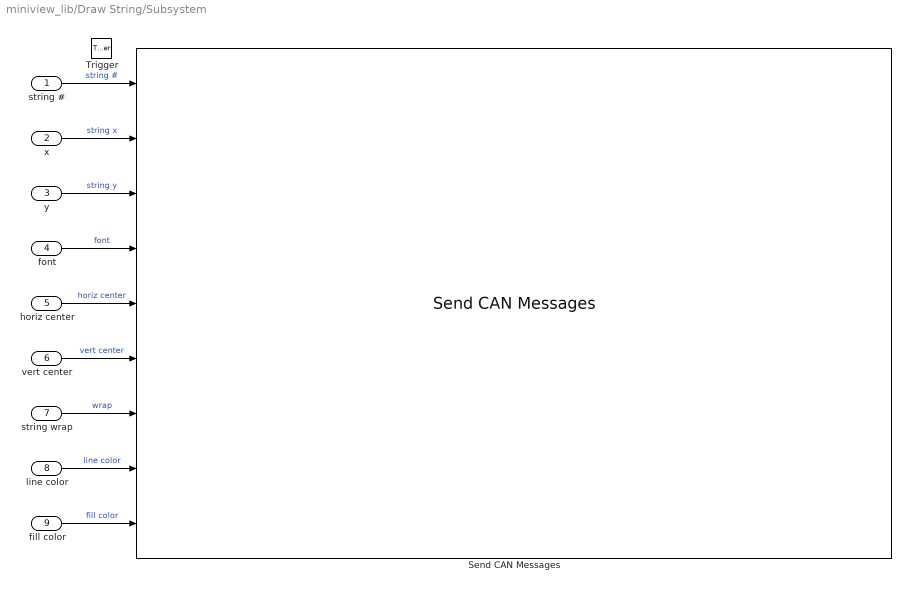
== system miniview_lib/Draw String/Subsystem ==
  string # : Inport
  x : Inport  Port=2
  y : Inport  Port=3
  font : Inport  Port=4
  horiz center : Inport  Port=5
  vert center : Inport  Port=6
  string wrap : Inport  Port=7
  line color : Inport  Port=8
  fill color : Inport  Port=9
  Trigger : TriggerPort  TriggerType=function-call
  Send CAN Messages : MotoHawk_lib/CAN Blocks/Send CAN Messages  bus=miniview_CAN_channel  msgl=miniview_draw_string  pace=-1  labelwires=on
  wires:
  y/1 -> Send CAN Messages/3  "string y"
  x/1 -> Send CAN Messages/2  "string x"
  string #/1 -> Send CAN Messages/1  "string #"
  font/1 -> Send CAN Messages/4  "font"
  horiz center/1 -> Send CAN Messages/5  "horiz center"
  string wrap/1 -> Send CAN Messages/7  "wrap"
  vert center/1 -> Send CAN Messages/6  "vert center"
  line color/1 -> Send CAN Messages/8  "line color"
  fill color/1 -> Send CAN Messages/9  "fill color"

== system miniview_lib/Draw Vline/Subsystem ==
  x : Inport
  y0 : Inport  Port=2
  y1 : Inport  Port=3
  line color : Inport  Port=4
  fill color : Inport  Port=5
  Trigger : TriggerPort  TriggerType=function-call
  Send CAN Messages : MotoHawk_lib/CAN Blocks/Send CAN Messages  bus=miniview_CAN_channel  msgl=miniview_draw_vline  pace=-1  labelwires=on
  wires:
  fill color/1 -> Send CAN Messages/5  "fill color"
  line color/1 -> Send CAN Messages/4  "line color"
  x/1 -> Send CAN Messages/1  "vline x"
  y0/1 -> Send CAN Messages/2  "vline y0"
  y1/1 -> Send CAN Messages/3  "vline y1"

== system miniview_lib/Menu Button/Subsystem ==
  Trigger : TriggerPort  TriggerType=function-call
  Read CAN Message : MotoHawk_lib/CAN Blocks/Read CAN Message  bus=miniview_CAN_channel  msg=miniview_button_menu  queue=1  slot='miniview_button_menu'  valid=off  stale=off  labelwires=on
  Signal Specification : simulink/Signal Attributes/Signal Specification  D=-1  Ts=-1  DataType=boolean  OutDataType=sfix(16)  OutScaling=2^0
      settings: SignalType=auto  SamplingMode=auto
  Signal Specification1 : simulink/Signal Attributes/Signal Specification  D=-1  Ts=-1  DataType=uint8  OutDataType=sfix(16)  OutScaling=2^0
      settings: SignalType=auto  SamplingMode=auto
  Out1 : Outport
  Out2 : Outport  Port=2
  wires:
  Signal Specification1/1 -> Out2/1  "menu count"
  Signal Specification/1 -> Out1/1  "menu asserted"
  Read CAN Message/2 -> Signal Specification1/1  "menu count"
  Read CAN Message/1 -> Signal Specification/1  "menu asserted"

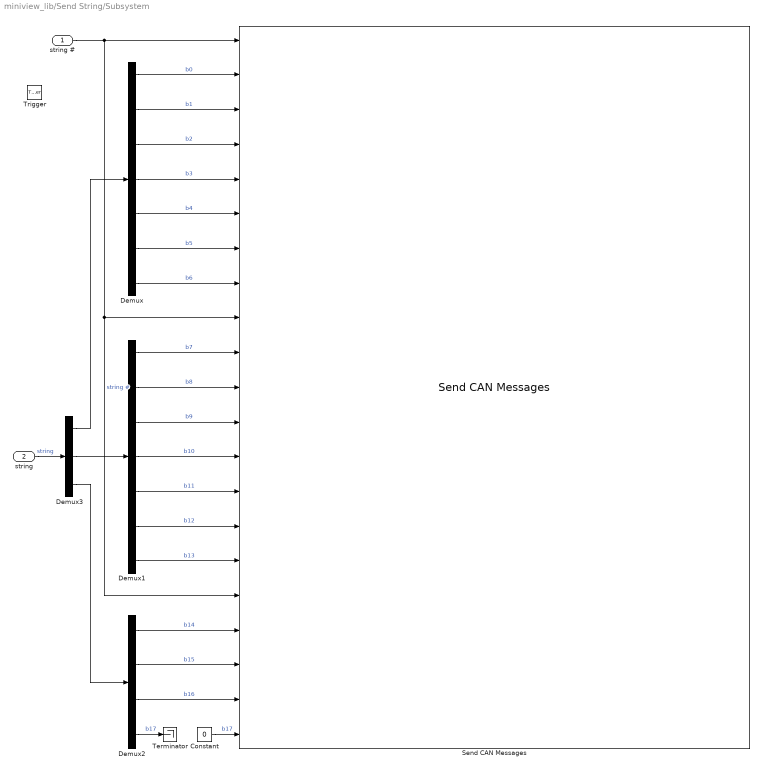
== system miniview_lib/Send String/Subsystem ==
  string # : Inport
  string : Inport  Port=2
  Trigger : TriggerPort  TriggerType=function-call
  Constant : Constant  Value=0
  Demux : Demux  Outputs=7
  Demux1 : Demux  Outputs=7
  Demux2 : Demux
  Demux3 : Demux  Outputs=[7 7 4]
  Send CAN Messages : MotoHawk_lib/CAN Blocks/Send CAN Messages  bus=miniview_CAN_channel  msgl=[miniview_string_xfer_page0 miniview_string_xfer_page1 miniview_string_xfer_page2]  pace=0  labelwires=on
  Terminator : Terminator
  wires:
  string #/1 -> Send CAN Messages/1, Send CAN Messages/17, Send CAN Messages/9  "string #"
  Demux/1 -> Send CAN Messages/2  "b0"
  Demux/2 -> Send CAN Messages/3  "b1"
  Demux/3 -> Send CAN Messages/4  "b2"
  Demux/4 -> Send CAN Messages/5  "b3"
  Demux/5 -> Send CAN Messages/6  "b4"
  Demux/6 -> Send CAN Messages/7  "b5"
  Demux/7 -> Send CAN Messages/8  "b6"
  Demux1/1 -> Send CAN Messages/10  "b7"
  Demux1/2 -> Send CAN Messages/11  "b8"
  Demux1/3 -> Send CAN Messages/12  "b9"
  Demux1/4 -> Send CAN Messages/13  "b10"
  Demux1/5 -> Send CAN Messages/14  "b11"
  Demux1/6 -> Send CAN Messages/15  "b12"
  Demux1/7 -> Send CAN Messages/16  "b13"
  Demux2/1 -> Send CAN Messages/18  "b14"
  Demux2/2 -> Send CAN Messages/19  "b15"
  Demux2/3 -> Send CAN Messages/20  "b16"
  string/1 -> Demux3/1  "string"
  Demux3/1 -> Demux/1
  Demux3/2 -> Demux1/1
  Demux3/3 -> Demux2/1
  Constant/1 -> Send CAN Messages/21  "b17"
  Demux2/4 -> Terminator/1  "b17"

== system miniview_lib/Send Substring (page 0)/Subsystem ==
  string # : Inport
  string : Inport  Port=2
  Trigger : TriggerPort  TriggerType=function-call
  Demux : Demux  Outputs=7
  Send CAN Messages : MotoHawk_lib/CAN Blocks/Send CAN Messages  bus=miniview_CAN_channel  msgl=miniview_string_xfer_page0  pace=0  labelwires=on
  wires:
  string/1 -> Demux/1  "string"
  Demux/7 -> Send CAN Messages/8  "b6"
  Demux/6 -> Send CAN Messages/7  "b5"
  Demux/5 -> Send CAN Messages/6  "b4"
  Demux/4 -> Send CAN Messages/5  "b3"
  Demux/3 -> Send CAN Messages/4  "b2"
  Demux/2 -> Send CAN Messages/3  "b1"
  Demux/1 -> Send CAN Messages/2  "b0"
  string #/1 -> Send CAN Messages/1  "string #"

== system miniview_lib/Send Substring (page 1)/Subsystem ==
  string # : Inport
  string : Inport  Port=2
  Trigger : TriggerPort  TriggerType=function-call
  Demux1 : Demux  Outputs=7
  Send CAN Messages : MotoHawk_lib/CAN Blocks/Send CAN Messages  bus=miniview_CAN_channel  msgl=miniview_string_xfer_page1  pace=0  labelwires=on
  wires:
  string #/1 -> Send CAN Messages/1  "string #"
  Demux1/1 -> Send CAN Messages/2  "b7"
  Demux1/2 -> Send CAN Messages/3  "b8"
  Demux1/3 -> Send CAN Messages/4  "b9"
  Demux1/4 -> Send CAN Messages/5  "b10"
  Demux1/5 -> Send CAN Messages/6  "b10"
  Demux1/6 -> Send CAN Messages/7  "b11"
  Demux1/7 -> Send CAN Messages/8  "b12"
  string/1 -> Demux1/1  "string"

== system miniview_lib/Send Substring (page 2)/Subsystem ==
  string # : Inport
  string : Inport  Port=2
  Trigger : TriggerPort  TriggerType=function-call
  Constant : Constant  Value=0
  Demux2 : Demux  Outputs=3
  Send CAN Messages : MotoHawk_lib/CAN Blocks/Send CAN Messages  bus=miniview_CAN_channel  msgl=miniview_string_xfer_page2  pace=0  labelwires=on
  wires:
  string #/1 -> Send CAN Messages/1  "string #"
  Demux2/1 -> Send CAN Messages/2  "b14"
  Demux2/2 -> Send CAN Messages/3  "b15"
  Demux2/3 -> Send CAN Messages/4  "b16"
  string/1 -> Demux2/1  "string"
  Constant/1 -> Send CAN Messages/5  "b17"

== system miniview_lib/Set GUI Mode/Subsystem ==
  mode : Inport
  Trigger : TriggerPort  TriggerType=function-call
  Send CAN Messages : MotoHawk_lib/CAN Blocks/Send CAN Messages  bus=miniview_CAN_channel  msgl=miniview_set_gui_mode  pace=-1  labelwires=on
  wires:
  mode/1 -> Send CAN Messages/1  "mode"

== system miniview_lib/Up Button/Subsystem ==
  Trigger : TriggerPort  TriggerType=function-call
  Read CAN Message : MotoHawk_lib/CAN Blocks/Read CAN Message  bus=miniview_CAN_channel  msg=miniview_button_up  queue=1  slot='miniview_button_up'  valid=off  stale=off  labelwires=on
  Signal Specification : simulink/Signal Attributes/Signal Specification  D=-1  Ts=-1  DataType=boolean  OutDataType=sfix(16)  OutScaling=2^0
      settings: SignalType=auto  SamplingMode=auto
  Signal Specification1 : simulink/Signal Attributes/Signal Specification  D=-1  Ts=-1  DataType=uint8  OutDataType=sfix(16)  OutScaling=2^0
      settings: SignalType=auto  SamplingMode=auto
  Out1 : Outport
  Out2 : Outport  Port=2
  wires:
  Read CAN Message/1 -> Signal Specification/1  "up asserted"
  Read CAN Message/2 -> Signal Specification1/1  "up count"
  Signal Specification/1 -> Out1/1  "up asserted"
  Signal Specification1/1 -> Out2/1  "up count"
